simulink library "lib_newData_range_check"  (R2023b)
settings: Solver=VariableStepAuto  StartTime=0.0  StopTime=10.0  RelTol=1e-3
settings Model: Creator=Administrator  LastModifiedBy=bowen
settings SolverCC: AlgebraicLoopSolver=TrustRegion
settings DebuggingCC: UnconnectedInputMsg=warning  UnconnectedOutputMsg=warning  UnconnectedLineMsg=warning
settings ModelReferenceCC: EnableRefExpFcnMdlSchedulingChecks=on

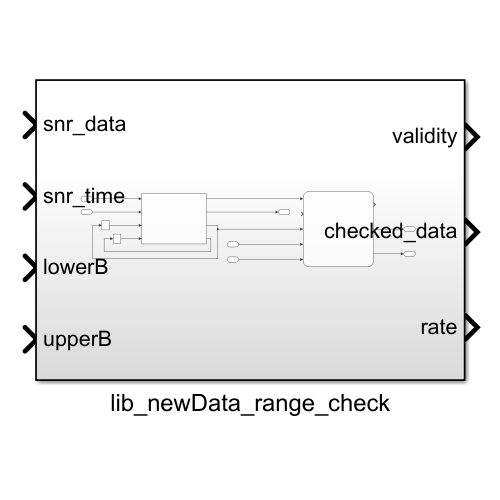
[thumbnail: Simulink's stored preview of the top-level diagram]
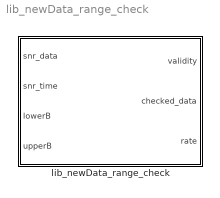
== system lib_newData_range_check ==
  lib_newData_range_check : Subsystem

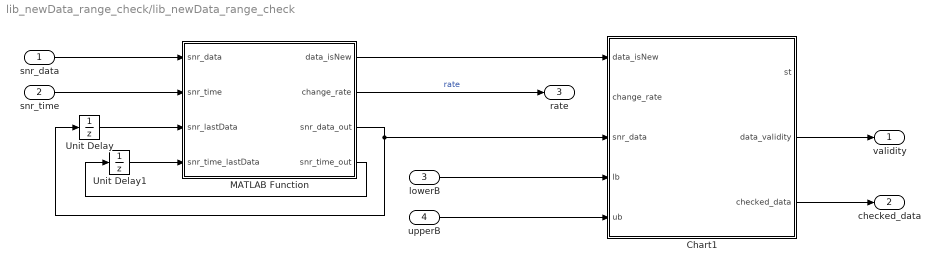
== system lib_newData_range_check/lib_newData_range_check ==
  snr_data : Inport  OutDataTypeStr=single
  snr_time : Inport  Port=2  OutDataTypeStr=single
  lowerB : Inport  Port=3  OutDataTypeStr=single
  upperB : Inport  Port=4  OutDataTypeStr=single
  Chart1 : Stateflow chart  TreatAsAtomicUnit=on
  MATLAB Function : MATLAB Function  TreatAsAtomicUnit=on
  Unit Delay : UnitDelay  SampleTime=-1  HasFrameUpgradeWarning=on
  Unit Delay1 : UnitDelay  SampleTime=-1  HasFrameUpgradeWarning=on
  validity : Outport
  checked_data : Outport  Port=2
  rate : Outport  Port=3
  wires:
  snr_time/1 -> MATLAB Function/2(snr_time)
  Unit Delay1/1 -> MATLAB Function/4(snr_time_lastData)
  Unit Delay/1 -> MATLAB Function/3(snr_lastData)
  MATLAB Function/1(data_isNew) -> Chart1/1(data_isNew)
  snr_data/1 -> MATLAB Function/1(snr_data)
  MATLAB Function/4(snr_time_out) -> Unit Delay1/1
  lowerB/1 -> Chart1/4(lb)
  upperB/1 -> Chart1/5(ub)
  MATLAB Function/2(change_rate) -> rate/1  "rate"
  MATLAB Function/3(snr_data_out) -> Unit Delay/1, Chart1/3(snr_data)
  Chart1/2(data_validity) -> validity/1
  Chart1/3(checked_data) -> checked_data/1

== stateflow chart lib_newData_range_check/Chart1 ==
  state No
    en:
    st = 0;
    data_validity = false;
    checked_data = snr_data;
    du:
    checked_data = snr_data;
  state possible1
    en:
    st = 1;
    checked_data = snr_data;
    du:
    checked_data = snr_data;
  note: ### consider add the rate check (2delta)
  state comfirmed
    en:
    st = 2;
    checked_data = snr_data;
    du:
    checked_data = snr_data;
  (default) -> No
  possible1 -> No [order 3] : after(0.1, sec)
  possible1 -> No [order 1] : [    ( data > ub ) ...
      |   || ( data < lb ) ]
  No -> (junction 6) : [data_isNew]
  (junction 6) -> possible1 : [    ( snr_data < ub) ...
      | && ( snr_data > lb) ]
  comfirmed -> possible1 : [( data > ub ) ...
      |   || ( data < lb )]
  possible1 -> (junction 13) [order 2] : [data_isNew]
  (junction 13) -> comfirmed : [   ( snr_data < ub) ...
      | && ( snr_data > lb) ]
  data: data_isNew input boolean; change_rate input double; snr_data input double; lb input double; ub input double; st output double; data_validity output boolean; checked_data output double

== matlab function lib_newData_range_check/MATLAB Function ==
  data: snr_data input single; snr_time input single; data_isNew output boolean; change_rate output; snr_lastData input single; snr_time_lastData input single; snr_data_out output single; snr_time_out output single
function [data_isNew, change_rate, snr_data_out, snr_time_out] = fcn(snr_data, snr_time, snr_lastData, snr_time_lastData)

data_isNew = false; 
snr_data_out = snr_lastData;
snr_time_out = snr_time_lastData;
change_rate = single(0);


if ( snr_time - snr_time_lastData )> 0.001     % sec
    data_isNew = true;   
    change_rate = (snr_data - snr_lastData) / (snr_time - snr_time_lastData);
    snr_data_out = snr_data;
    snr_time_out = snr_time;
end
